simulink model "A3VSM390"  (R2022a)
settings: Solver=ode14x  StartTime=0  StopTime=Sim.tend  FixedStep=0.000125  RelTol=4e-4
values from neighbouring files (symbols this model uses):
  center_line_status = parameterset.center_line_status    [sim3run_390.m]
  ControlSampleTime = 1/8000    (= 0.000125)    [sim3run_390.m]
  k_ring1 = 1    [sim3run_390.m]
  k_ring2 = 1    [sim3run_390.m]
  load_start_factor = 1    [prm3var_390.m]    (also in simu3_826.m = 0.9; simu3_827.m = 0.9)
  lower_line_status = parameterset.lower_line_status    [sim3run_390.m]
  mZC = 3    [sim3run_390.m]
undefined symbols (not defined in the file or in its folder): Event, General, InfBus, Li, parameterset, prm_vsm, pu_vsm, TrG, VSM
libraries: fl_lib x92, nesl_utility x69, ee_lib x36, spsPower3phInstantaneousLib x5, simulink x2, eeTransforms x1
(part 1 of 3)
settings Model: Creator=e2n052  LastModifiedBy=uk062294
settings SolverCC: AlgebraicLoopSolver=TrustRegion
settings DataIOCC: ReturnWorkspaceOutputs=off
settings DebuggingCC: UnconnectedInputMsg=warning  UnconnectedOutputMsg=warning  UnconnectedLineMsg=warning  ArithmeticOperatorsInVariantConditions=warning
settings SFSimCC: SimUseLocalCustomCode=off  CustomCodeUndefinedFunction=UseInterfaceOnly
settings RTWCC: RTWUseLocalCustomCode=off  DLArmComputeVersion=19.05

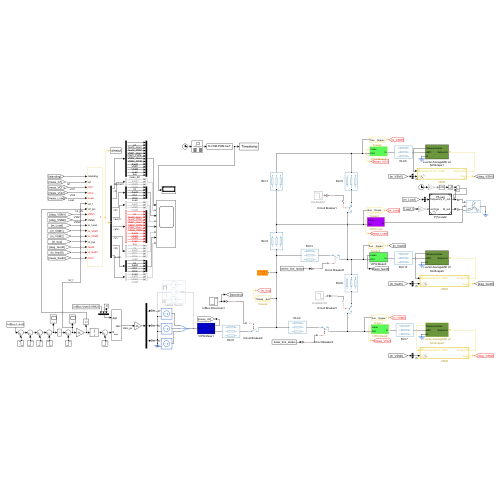
[thumbnail: Simulink's stored preview of the top-level diagram]
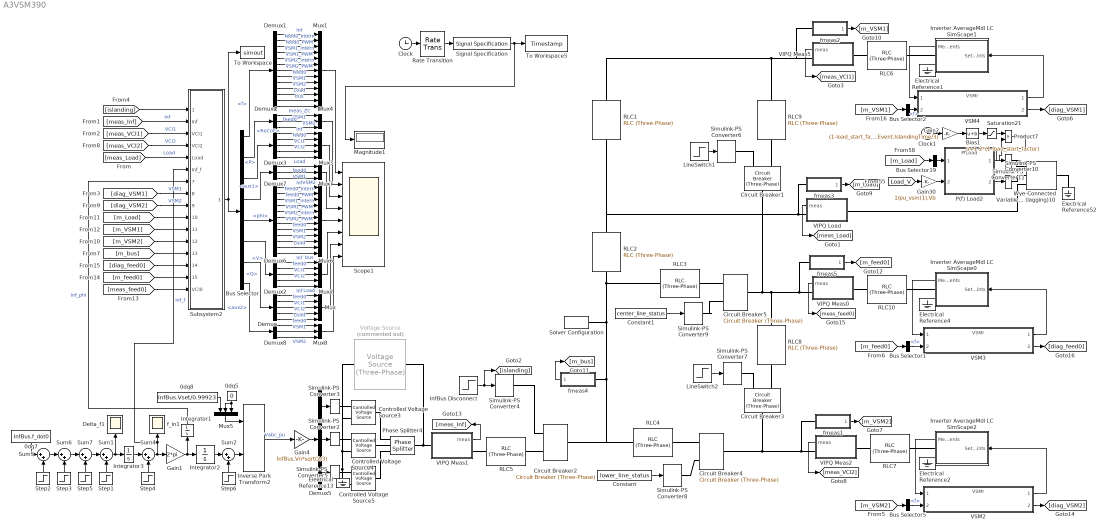
== system A3VSM390 ==
  0dq5 : Constant  Value=0
  0dq7 : Constant  Value=InfBus.f_dot0
  0dq8 : Constant  Value=InfBus.Vset/0.99923
  Bias1 : Bias  Bias=1-2*(1-load_start_factor)  SaturateOnIntegerOverflow=off
  Bus Selector : BusSelector  OutputSignals=f,RoCoF,P,aux1,phi,V,Q,aux2
  Bus Selector1 : BusSelector  OutputSignals=f
  Bus Selector19 : BusSelector  OutputSignals=f  OutputAsBus=on
  Bus Selector2 : BusSelector  OutputSignals=f
  Bus Selector5 : BusSelector  OutputSignals=f
  Circuit Breaker{1,3..5} (4 alike) : ee_lib/Switches & Breakers/Circuit Breaker (Three-Phase)  R_closed=0.0001 Ohm  G_open=1e-6 1/Ohm  threshold=0.5 V  breaker_behavior=ee.enum.switches.breakerBehavior.zeroCrossingEnable
      settings: InternalSimscapePortConfiguration="{\"Bottom\":[],\"Left\":[{\"id\":\"vT\",\"label\":\"vT\",\"type\":\"input\"},{\"id\":\"N1\",\"label\":\"~1\",\"type\":\"foundation.electrical.three_phase\"}],\"Right\":[{\"id\":\"N2\",\"label\":\"~2\",\"type\":\"foundation.electrical.three_phase\"}],\"Top\":[]}"
  Circuit Breaker2 : ee_lib/Switches & Breakers/Circuit Breaker (Three-Phase)  R_closed=0.001 Ohm  G_open=1e-6 1/Ohm  threshold=0.5 V  breaker_behavior=ee.enum.switches.breakerBehavior.zeroCrossingEnable
      settings: InternalSimscapePortConfiguration="{\"Bottom\":[],\"Left\":[{\"id\":\"vT\",\"label\":\"vT\",\"type\":\"input\"},{\"id\":\"N1\",\"label\":\"~1\",\"type\":\"foundation.electrical.three_phase\"}],\"Right\":[{\"id\":\"N2\",\"label\":\"~2\",\"type\":\"foundation.electrical.three_phase\"}],\"Top\":[]}"
  Clock : Clock
  Clock1 : Clock
  Constant : Constant  Value=lower_line_status
  Constant1 : Constant  Value=center_line_status
  Controlled Voltage Source3 : fl_lib/Electrical/Electrical Sources/Controlled Voltage Source
  Controlled Voltage Source4 : fl_lib/Electrical/Electrical Sources/Controlled Voltage Source
  Controlled Voltage Source5 : fl_lib/Electrical/Electrical Sources/Controlled Voltage Source
  Delta_f1 : Scope
  Demux : Demux  Outputs=5
  Demux1 : Demux  Outputs=13
  Demux2 : Demux  Outputs=5
  Demux3 : Demux  Outputs=5
  Demux{4..5,7..8} (4 alike) : Demux  Outputs=3
  Demux6 : Demux  Outputs=12
  Electrical Reference{1..2,4,13,52} (5 alike) : fl_lib/Electrical/Electrical Elements/Electrical Reference
  Gain1 : Gain  Gain=2*pi
  Gain2 : Gain  Gain=(1-load_start_factor)/(parameterset.Event.IslandingTime/3)
  Gain30 : Gain  Gain=1/pu_vsm(1).Vb
  Gain4 : Gain  Gain=InfBus.Vn*sqrt(2/3)
  InfBus Disconnect : Step  Time=Event.IslandingTime  SampleTime=0
  Integrator1 : Integrator  InitialCondition=0+prm_vsm{19,2}  WrappedStateUpperValue=2*pi  WrappedStateLowerValue=0
  Integrator2 : Integrator  InitialCondition=pi/2+prm_vsm{19,2}  WrappedStateUpperValue=2*pi  WrappedStateLowerValue=0
  Integrator3 : Integrator  InitialCondition=InfBus.f_init-InfBus.fn
  Inverse Park Transform2 : eeTransforms/Inverse Park Transform  AxisAlignment=Q-axis  PowerInvariant=off
  Inverter AverageMdl LC SimScape0 : Subsystem  VariantControl=PMXXF33C  mask{L1=prm_vsm{40,3}, R_L1=prm_vsm{43,3}, C1=prm_vsm{42,3}, R_C1=prm_vsm{45,3}}
      mask prompts: L1 "Inductance L1 [H]"; R_L1 "Resistance of L1 [Ohm]"; C1 "Capacitance C1 [F]"; R_C1 "Parallel resistance of C1 [Ohm]"
      mask DialogControl GrpLC Prompt: LC(L)(C)-Filter
  Inverter AverageMdl LC SimScape1 : Subsystem  VariantControl=PMXXF33C  mask{L1=prm_vsm{40,4}, R_L1=prm_vsm{43,4}, C1=prm_vsm{42,4}, R_C1=prm_vsm{45,4}}
      mask prompts: L1 "Inductance L1 [H]"; R_L1 "Resistance of L1 [Ohm]"; C1 "Capacitance C1 [F]"; R_C1 "Parallel resistance of C1 [Ohm]"
      mask DialogControl GrpLC Prompt: LC(L)(C)-Filter
  Inverter AverageMdl LC SimScape2 : Subsystem  VariantControl=PMXXF33C  mask{L1=prm_vsm{40,2}, R_L1=prm_vsm{43,2}, C1=prm_vsm{42,2}, R_C1=prm_vsm{45,2}}
      mask prompts: L1 "Inductance L1 [H]"; R_L1 "Resistance of L1 [Ohm]"; C1 "Capacitance C1 [F]"; R_C1 "Parallel resistance of C1 [Ohm]"
      mask DialogControl GrpLC Prompt: LC(L)(C)-Filter
  "LineSwitch1 " : Step  Time=Event.ring1_switch_time  Before=Event.ring1_switch_direction  After=1-Event.ring1_switch_direction  SampleTime=0
  LineSwitch2 : Step  Time=Event.ring2_switch_time  Before=Event.ring2_switch_direction  After=1-Event.ring2_switch_direction  SampleTime=0
  Magnitude1 : Display
  Mux : Mux  Inputs=5
  Mux1 : Mux  Inputs=13
  Mux2 : Mux  Inputs=5
  Mux3 : Mux  Inputs=5
  Mux{4..5,7..8} (4 alike) : Mux  Inputs=3
  Mux6 : Mux  Inputs=12
  P(f) Load2 : ModelReference  ModelNameDialog=PfLoad.slx  UsingDefaultArgumentValue=0  SimulationMode=Normal  ModelReferenceVersion=11.283
  Phase Splitter4 : ee_lib/Connectors & References/Phase Splitter
  Product7 : Product
  RLC1 : ee_lib/Passive/RLC Assemblies/RLC (Three-Phase)  component_structure=4  R=Li.length*Li.R Ohm  L=Li.length*Li.L H  C=1e-6 F  R_parasitic=1e-6 Ohm  G_parasitic=1e-6 1/Ohm  IL_specify=on  IL_priority=High  IL=[0, 0, 0] A  IL_nominal_specify=off  IL_nominal_unit=A  IL_nominal_value=1  VC_specify=on  VC_priority=High  VC=[0, 0, 0] V  VC_nominal_specify=off  VC_nominal_unit=V  VC_nominal_value=1
      settings: InternalSimscapePortConfiguration="{\"Bottom\":[],\"Left\":[{\"id\":\"N1\",\"label\":\"~1\",\"type\":\"foundation.electrical.three_phase\"}],\"Right\":[{\"id\":\"N2\",\"label\":\"~2\",\"type\":\"foundation.electrical.three_phase\"}],\"Top\":[]}"
  RLC10 : ee_lib/Passive/RLC Assemblies/RLC (Three-Phase)  component_structure=4  R=prm_vsm{44,3} Ohm  L=prm_vsm{41,3} H  C=1e-6 F  R_parasitic=1e-6 Ohm  G_parasitic=1e-6 1/Ohm  IL_specify=on  IL_priority=High  IL=[0, 0, 0] A  IL_nominal_specify=off  IL_nominal_unit=A  IL_nominal_value=1  VC_specify=on  VC_priority=High  VC=[0, 0, 0] V  VC_nominal_specify=off  VC_nominal_unit=V  VC_nominal_value=1
      settings: InternalSimscapePortConfiguration="{\"Bottom\":[],\"Left\":[{\"id\":\"N1\",\"label\":\"~1\",\"type\":\"foundation.electrical.three_phase\"}],\"Right\":[{\"id\":\"N2\",\"label\":\"~2\",\"type\":\"foundation.electrical.three_phase\"}],\"Top\":[]}"
  RLC2 : ee_lib/Passive/RLC Assemblies/RLC (Three-Phase)  component_structure=4  R=Li.length*Li.R Ohm  L=Li.length*Li.L H  C=1e-6 F  R_parasitic=1e-6 Ohm  G_parasitic=1e-6 1/Ohm  IL_specify=on  IL_priority=High  IL=[0, 0, 0] A  IL_nominal_specify=off  IL_nominal_unit=A  IL_nominal_value=1  VC_specify=on  VC_priority=High  VC=[0, 0, 0] V  VC_nominal_specify=off  VC_nominal_unit=V  VC_nominal_value=1
      settings: InternalSimscapePortConfiguration="{\"Bottom\":[],\"Left\":[{\"id\":\"N1\",\"label\":\"~1\",\"type\":\"foundation.electrical.three_phase\"}],\"Right\":[{\"id\":\"N2\",\"label\":\"~2\",\"type\":\"foundation.electrical.three_phase\"}],\"Top\":[]}"
  RLC3 : ee_lib/Passive/RLC Assemblies/RLC (Three-Phase)  component_structure=4  R=2*Li.length*Li.R Ohm  L=2*Li.length*Li.L H  C=1e-6 F  R_parasitic=1e-6 Ohm  G_parasitic=1e-6 1/Ohm  IL_specify=on  IL_priority=High  IL=[0, 0, 0] A  IL_nominal_specify=off  IL_nominal_unit=A  IL_nominal_value=1  VC_specify=on  VC_priority=High  VC=[0, 0, 0] V  VC_nominal_specify=off  VC_nominal_unit=V  VC_nominal_value=1
      settings: InternalSimscapePortConfiguration="{\"Bottom\":[],\"Left\":[{\"id\":\"N1\",\"label\":\"~1\",\"type\":\"foundation.electrical.three_phase\"}],\"Right\":[{\"id\":\"N2\",\"label\":\"~2\",\"type\":\"foundation.electrical.three_phase\"}],\"Top\":[]}"
  RLC4 : ee_lib/Passive/RLC Assemblies/RLC (Three-Phase)  component_structure=4  R=2*Li.length*Li.R Ohm  L=2*Li.length*Li.L H  C=1e-6 F  R_parasitic=1e-6 Ohm  G_parasitic=1e-6 1/Ohm  IL_specify=on  IL_priority=High  IL=[0, 0, 0] A  IL_nominal_specify=off  IL_nominal_unit=A  IL_nominal_value=1  VC_specify=on  VC_priority=High  VC=[0, 0, 0] V  VC_nominal_specify=off  VC_nominal_unit=V  VC_nominal_value=1
      settings: InternalSimscapePortConfiguration="{\"Bottom\":[],\"Left\":[{\"id\":\"N1\",\"label\":\"~1\",\"type\":\"foundation.electrical.three_phase\"}],\"Right\":[{\"id\":\"N2\",\"label\":\"~2\",\"type\":\"foundation.electrical.three_phase\"}],\"Top\":[]}"
  RLC5 : ee_lib/Passive/RLC Assemblies/RLC (Three-Phase)  component_structure=4  R=TrG.R Ohm  L=TrG.L H  C=1e-6 F  R_parasitic=1e-6 Ohm  G_parasitic=1e-6 1/Ohm  IL_specify=on  IL_priority=High  IL=[0, 0, 0] A  IL_nominal_specify=off  IL_nominal_unit=A  IL_nominal_value=1  VC_specify=on  VC_priority=High  VC=[0, 0, 0] V  VC_nominal_specify=off  VC_nominal_unit=V  VC_nominal_value=1
      settings: InternalSimscapePortConfiguration="{\"Bottom\":[],\"Left\":[{\"id\":\"N1\",\"label\":\"~1\",\"type\":\"foundation.electrical.three_phase\"}],\"Right\":[{\"id\":\"N2\",\"label\":\"~2\",\"type\":\"foundation.electrical.three_phase\"}],\"Top\":[]}"
  RLC6 : ee_lib/Passive/RLC Assemblies/RLC (Three-Phase)  component_structure=4  R=prm_vsm{44,4} Ohm  L=prm_vsm{41,4} H  C=1e-6 F  R_parasitic=1e-6 Ohm  G_parasitic=1e-6 1/Ohm  IL_specify=on  IL_priority=High  IL=[0, 0, 0] A  IL_nominal_specify=off  IL_nominal_unit=A  IL_nominal_value=1  VC_specify=on  VC_priority=High  VC=[0, 0, 0] V  VC_nominal_specify=off  VC_nominal_unit=V  VC_nominal_value=1
      settings: InternalSimscapePortConfiguration="{\"Bottom\":[],\"Left\":[{\"id\":\"N1\",\"label\":\"~1\",\"type\":\"foundation.electrical.three_phase\"}],\"Right\":[{\"id\":\"N2\",\"label\":\"~2\",\"type\":\"foundation.electrical.three_phase\"}],\"Top\":[]}"
  RLC7 : ee_lib/Passive/RLC Assemblies/RLC (Three-Phase)  component_structure=4  R=prm_vsm{44,2} Ohm  L=prm_vsm{41,2} H  C=1e-6 F  R_parasitic=1e-6 Ohm  G_parasitic=1e-6 1/Ohm  IL_specify=on  IL_priority=High  IL=[0, 0, 0] A  IL_nominal_specify=off  IL_nominal_unit=A  IL_nominal_value=1  VC_specify=on  VC_priority=High  VC=[0, 0, 0] V  VC_nominal_specify=off  VC_nominal_unit=V  VC_nominal_value=1
      settings: InternalSimscapePortConfiguration="{\"Bottom\":[],\"Left\":[{\"id\":\"N1\",\"label\":\"~1\",\"type\":\"foundation.electrical.three_phase\"}],\"Right\":[{\"id\":\"N2\",\"label\":\"~2\",\"type\":\"foundation.electrical.three_phase\"}],\"Top\":[]}"
  RLC8 : ee_lib/Passive/RLC Assemblies/RLC (Three-Phase)  component_structure=4  R=k_ring2*Li.length*Li.R Ohm  L=k_ring2*Li.length*Li.L H  C=1e-6 F  R_parasitic=1e-6 Ohm  G_parasitic=1e-6 1/Ohm  IL_specify=on  IL_priority=High  IL=[0, 0, 0] A  IL_nominal_specify=off  IL_nominal_unit=A  IL_nominal_value=1  VC_specify=on  VC_priority=High  VC=[0, 0, 0] V  VC_nominal_specify=off  VC_nominal_unit=V  VC_nominal_value=1
      settings: InternalSimscapePortConfiguration="{\"Bottom\":[],\"Left\":[{\"id\":\"N1\",\"label\":\"~1\",\"type\":\"foundation.electrical.three_phase\"}],\"Right\":[{\"id\":\"N2\",\"label\":\"~2\",\"type\":\"foundation.electrical.three_phase\"}],\"Top\":[]}"
  RLC9 : ee_lib/Passive/RLC Assemblies/RLC (Three-Phase)  component_structure=4  R=k_ring1*Li.length*Li.R Ohm  L=k_ring1*Li.length*Li.L H  C=1e-6 F  R_parasitic=1e-6 Ohm  G_parasitic=1e-6 1/Ohm  IL_specify=on  IL_priority=High  IL=[0, 0, 0] A  IL_nominal_specify=off  IL_nominal_unit=A  IL_nominal_value=1  VC_specify=on  VC_priority=High  VC=[0, 0, 0] V  VC_nominal_specify=off  VC_nominal_unit=V  VC_nominal_value=1
      settings: InternalSimscapePortConfiguration="{\"Bottom\":[],\"Left\":[{\"id\":\"N1\",\"label\":\"~1\",\"type\":\"foundation.electrical.three_phase\"}],\"Right\":[{\"id\":\"N2\",\"label\":\"~2\",\"type\":\"foundation.electrical.three_phase\"}],\"Top\":[]}"
  Rate Transition : RateTransition  OutPortSampleTimeOpt=Inherit
  Saturation21 : Saturate  UpperLimit=1  LowerLimit=load_start_factor
  Scope1 : Scope  NumInputPorts=8
  Signal Specification : SignalSpecification  SampleTime=VSM.PWM.tauT
  Simulink-PS Converter{4,6..11} (7 alike) : nesl_utility/Simulink-PS Converter  PhysicalDomain=network_engine_domain  SubClassName=ps_input  LeftPortType=input  RightPortType=output  PseudoPeriodic=off  Frequencies=[]  NoiseDistribution=none  NoiseParameters=[]  Unit=1  AffineConversion=off  FilteringAndDerivatives=zero  SimscapeFilterOrder=1  InputFilterTimeConstant=0.001  UdotUserProvided=1
  Simulink-PS Converter2 : nesl_utility/Simulink-PS Converter  PhysicalDomain=network_engine_domain  SubClassName=ps_input  LeftPortType=input  RightPortType=output  PseudoPeriodic=off  Frequencies=[]  NoiseDistribution=none  NoiseParameters=[]  Unit=V  AffineConversion=off  FilteringAndDerivatives=filter  SimscapeFilterOrder=1  InputFilterTimeConstant=T_PSconv  UdotUserProvided=2
  Simulink-PS Converter3 : nesl_utility/Simulink-PS Converter  PhysicalDomain=network_engine_domain  SubClassName=ps_input  LeftPortType=input  RightPortType=output  PseudoPeriodic=off  Frequencies=[]  NoiseDistribution=none  NoiseParameters=[]  Unit=V  AffineConversion=off  FilteringAndDerivatives=filter  SimscapeFilterOrder=1  InputFilterTimeConstant=T_PSconv  UdotUserProvided=2
  Simulink-PS Converter5 : nesl_utility/Simulink-PS Converter  PhysicalDomain=network_engine_domain  SubClassName=ps_input  LeftPortType=input  RightPortType=output  PseudoPeriodic=off  Frequencies=[]  NoiseDistribution=none  NoiseParameters=[]  Unit=V  AffineConversion=off  FilteringAndDerivatives=filter  SimscapeFilterOrder=1  InputFilterTimeConstant=T_PSconv  UdotUserProvided=2
  Solver Configuration : nesl_utility/Solver Configuration  PhysicalDomain=network_engine_domain  SubClassName=solver  LeftPortType=input  RightPortType=generic  Tones=[]  Harmonics=[]  SimulateNoise=off  Profile=off  UseLocalSampling=off  EnableSwitchedLinearOptims=on  FrequencyDomain=off  UseCCode=off  RelTol=0.001  AbsTol=1e-06  MinStep=1e-09  ToWorkspace=off  RevertToSquareIcSolve=off  NumHomotopyIterations=100  PhasorMode=off  PhasorModeNumHarmonics=1  ConsistencySolver=NEWTON_FTOL  IndexReductionMethod=DerivativeReplacement  DoDC=off  ResidualTolerance=1e-09  ConsistencyTolSource=GLOBAL  ConsistencyAbsTol=0.001  ConsistencyRelTol=0.001  ConsistencyTolFactor=0.001  UseLocalSolver=on  LocalSolverChoice=NE_BACKWARD_EULER_ADVANCER  ResolveIndetEquations=on  FunctionEvalNumThread=1  LocalSolverSampleTime=1/8e3  DoFixedCost=on  MaxNonlinIter=3  MaxModeIter=2  ComputeImpulses=off  ImpulseIterations=2  LinearAlgebra=Sparse  LinearAlgebraNumThread=0  EquationFormulation=NE_TIME_EF  DelaysMemoryBudget=1024  AutomaticFiltering=off  FilteringTimeConstant=0.001  PartitionStorageMethod=AS_NEEDED  PartitionMemoryBudget=1024  PartitionMethod=FAST  MultibodyUseLocalSolver=off  MultibodyLocalSolverChoice=ODE1  MultibodyLocalSolverSampleTime=0.001
  Step1 : Step  Time=InfBus.t_fd4  After=InfBus.f_dot4-InfBus.f_dot3  SampleTime=0
  Step2 : Step  Time=InfBus.t_fd1  After=InfBus.f_dot1-InfBus.f_dot0  SampleTime=0
  Step3 : Step  Time=InfBus.t_fd2  After=InfBus.f_dot2-InfBus.f_dot1  SampleTime=0
  Step4 : Step  Time=InfBus.t_f1  Before=InfBus.fn  After=InfBus.f1  SampleTime=0
  Step5 : Step  Time=InfBus.t_fd3  After=InfBus.f_dot3-InfBus.f_dot2  SampleTime=0
  Step6 : Step  Time=InfBus.t_theta1  After=InfBus.delta_theta1  SampleTime=0
  Subsystem2 : Subsystem
  Sum{1..2,4..7} (6 alike) : Sum  Inputs=|++
  To Workspace : ToWorkspace  VariableName=simout  SampleTime=-1
  To Workspace5 : ToWorkspace  VariableName=Timestamp  SampleTime=-1
  VIPQ Load : Subsystem
  VIPQ Meas0 : Subsystem
  VIPQ Meas1 : Subsystem
  VIPQ Meas2 : Subsystem
  VIPQ Meas5 : Subsystem
  VSM2 : ModelReference  ModelNameDialog=VSMr.slx  UsingDefaultArgumentValue=0  SimulationMode=Normal  ModelReferenceVersion=8.11
  VSM3 : ModelReference  ModelNameDialog=VSMr.slx  UsingDefaultArgumentValue=0  SimulationMode=Normal  ModelReferenceVersion=8.11
  VSM4 : ModelReference  ModelNameDialog=VSMr.slx  UsingDefaultArgumentValue=0  SimulationMode=Normal  ModelReferenceVersion=8.11
  Voltage Source : ee_lib/Sources/Voltage Source (Three-Phase)  Commented=on  vline_rms=InfBus.Vn*InfBus.Vset V  shift=pi/2+VSM.VSM.Phi0-pi/2*0.12 rad  freq=InfBus.fn Hz  impedance_option=0  SShortCircuit=500e6 V*A  XR=10  R=0.01 Ohm  L=3.97e-4 H  harmonic_option=0  harmonic_orders=[5, 7, 11, 13]  harmonic_ratios=[0.1, 0.1, 0.1, 0.1]  G_parasitic=0 1/Ohm  I_specify=off  I_priority=None  I=[ 0 0 0 ] A  I_nominal_specify=off  I_nominal_unit=A  I_nominal_value=1
  Wye-Connected Variable Load (lagging)10 : ee_lib/Passive/RLC Assemblies/Wye-Connected Variable Load (lagging)  VRated=int_sup_vol1 V  FRated=50 Hz  Pmin=10 W  Qmin=10 A*V  G_parasitic=1e-6 1/Ohm  I_specify=off  I_priority=None  I=[0, 0, 0] A  I_nominal_specify=off  I_nominal_unit=A  I_nominal_value=1  Phi_specify=off  Phi_priority=None  Phi=[0, 0, 0] Wb  Phi_nominal_specify=off  Phi_nominal_unit=Wb  Phi_nominal_value=1
      settings: InternalSimscapePortConfiguration="{\"Bottom\":[],\"Left\":[{\"id\":\"P\",\"label\":\"P\",\"type\":\"input\"},{\"id\":\"Q\",\"label\":\"Q\",\"type\":\"input\"},{\"id\":\"N\",\"label\":\"~\",\"type\":\"foundation.electrical.three_phase\"}],\"Right\":[{\"id\":\"n\",\"label\":\"n\",\"type\":\"foundation.electrical.electrical\"}],\"Top\":[]}"
  f_in1 : Scope
  fmeas{1..5} (5 alike) : Subsystem  ReferencedSubsystem=f_meas
  wires:
  InfBus Disconnect/1 -> [islanding], Simulink-PS Converter4/1
  Bus Selector/7 -> Demux/1  "<Q>"
  Bus Selector/3 -> Demux3/1  "<P>"
  Demux3/1 -> Mux3/1  "Inf"
  Demux3/3 -> Mux3/3  "VCI1"
  Demux3/4 -> Mux3/4  "VCI2"
  Bus Selector/6 -> Demux2/1  "<V>"
  Demux2/4 -> Mux2/4  "VCI2"
  Demux2/3 -> Mux2/3  "VCI1"
  Demux2/1 -> Mux2/1  "Inf"
  Bus Selector/1 -> Demux1/1  "<f>"
  Demux1/1 -> Mux1/1  "Inf"
  Demux1/4 -> Mux1/4  "VSM1_intern"
  Demux1/5 -> Mux1/5  "VSM1_PWM"
  Demux/4 -> Mux/4  "VCI2"
  Demux/3 -> Mux/3  "VCI1"
  Demux/1 -> Mux/1  "Inf"
  Inverter AverageMdl LC SimScape1/1(Measurements) -> VSM4/1
  Subsystem2/1(Out5) -> Bus Selector/1, To Workspace/1
  VIPQ Meas5/1(meas) -> [meas_VCI1]
  VIPQ Meas1/1(meas) -> [meas_Inf]
  Clock/1 -> Rate Transition/1
  Sum5/1 -> Sum6/1
  Step2/1 -> Sum5/2
  Step5/1 -> Sum7/2
  Gain4/1 -> Demux5/1
  Demux5/3 -> Simulink-PS Converter5/1
  Demux5/2 -> Simulink-PS Converter2/1
  Mux5/1 -> Inverse Park Transform2/1
  Step3/1 -> Sum6/2
  Inverse Park Transform2/1 -> Gain4/1  "Vabc_pu"
  0dq7/1 -> Sum5/1
  Integrator3/1 -> Sum4/1
  0dq5/1 -> Mux5/2, Mux5/3
  Gain1/1 -> Integrator1/1, Integrator2/1
  Sum6/1 -> Sum7/1
  Step1/1 -> Sum1/2
  Sum7/1 -> Sum1/1
  Sum1/1 -> Integrator3/1, Delta_f1/1
  Demux6/4 -> Mux6/4  "VSM1_intern"
  Demux6/5 -> Mux6/5  "VSM1_PWM"
  Demux6/1 -> Mux6/1  "Inf"
  Bus Selector/5 -> Demux6/1  "<phi>"
  Mux1/1 -> Scope1/1
  Mux6/1 -> Scope1/5
  Mux3/1 -> Scope1/3
  Mux/1 -> Scope1/7
  Mux2/1 -> Scope1/6
  Inverter AverageMdl LC SimScape2/1(Measurements) -> VSM2/1
  VIPQ Meas2/1(meas) -> [meas_VCI2]
  Demux2/5 -> Mux2/5  "Load"
  Demux/5 -> Mux/5  "Load"
  Demux3/5 -> Mux3/5  "Load"
  Demux6/6 -> Mux6/6  "VSM2_intern"
  Demux1/6 -> Mux1/6  "VSM2_intern"
  "LineSwitch1 "/1 -> Simulink-PS Converter6/1
  VSM2/2 -> [diag_VSM2]
  VIPQ Load/1(meas) -> [meas_Load]
  VSM4/2 -> [diag_VSM1]
  Demux1/7 -> Mux1/7  "VSM2_PWM"
  Demux1/9 -> Mux1/9  "VSM1"
  Demux1/10 -> Mux1/10  "VSM2"
  Demux1/11 -> Mux1/11  "Load"
  Demux6/7 -> Mux6/7  "VSM2_PWM"
  Demux6/9 -> Mux6/9  "VSM1"
  Demux6/10 -> Mux6/10  "VSM2"
  [islanding] -> Subsystem2/1(Islanding)
  [meas_Inf] -> Subsystem2/2(Inf)  "Inf"
  [meas_VCI1] -> Subsystem2/3(VCI1)  "VCI1"
  [meas_VCI2] -> Subsystem2/4(VCI2)  "VCI2"
  [meas_Load] -> Subsystem2/5(Load)  "Load"
  Sum4/1 -> Subsystem2/6(Inf_f), f_in1/1, Gain1/1  "Inf_f"
  Integrator1/1 -> Subsystem2/7(Inf_phi)  "Inf_phi"
  [diag_VSM1] -> Subsystem2/8(VSM1)  "VSM1"
  [diag_VSM2] -> Subsystem2/9(VSM2)  "VSM2"
  [m_Load] -> Subsystem2/10(m_Load)
  [m_VSM1] -> Subsystem2/11(m_VSM1)
  Bus Selector/4 -> Demux7/1  "<aux1>"
  Bus Selector/8 -> Demux8/1  "<aux2>"
  0dq8/1 -> Mux5/1
  Demux5/1 -> Simulink-PS Converter3/1
  Integrator2/1 -> Sum2/1
  [m_VSM2] -> Subsystem2/12(m_VSM2)
  Demux1/12 -> Mux1/12  "bus"
  Demux1/13 -> Mux1/13  "meas_ZC"
  Demux6/11 -> Mux6/11  "Load"
  fmeas1/1 -> [m_VSM2]
  fmeas2/1 -> [m_VSM1]
  fmeas4/1 -> [m_bus]
  fmeas3/1 -> [m_Load]
  Demux6/12 -> Mux6/12  "bus"
  [m_bus] -> Subsystem2/13(m_bus)
  Step4/1 -> Sum4/2
  LineSwitch2/1 -> Simulink-PS Converter7/1
  Inverter AverageMdl LC SimScape0/1(Measurements) -> VSM3/1
  VIPQ Meas0/1(meas) -> [meas_feed0]
  fmeas5/1 -> [m_feed0]
  VSM3/2 -> [diag_feed0]
  [m_feed0] -> Subsystem2/15(m_feed0)
  Demux1/8 -> Mux1/8  "feed0"
  Demux1/3 -> Mux1/3  "feed0_PWM"
  Demux1/2 -> Mux1/2  "feed0_intern"
  Demux6/2 -> Mux6/2  "feed0_intern"
  Demux6/3 -> Mux6/3  "feed0_PWM"
  Demux6/8 -> Mux6/8  "feed0"
  Demux3/2 -> Mux3/2  "feed0"
  Demux/2 -> Mux/2  "feed0"
  Demux2/2 -> Mux2/2  "feed0"
  [diag_feed0] -> Subsystem2/14(feed0)
  [meas_feed0] -> Subsystem2/16(VCI0)
  Demux7/1 -> Mux7/1  "feed0"
  Demux7/2 -> Mux7/2  "VSM1"
  Demux7/3 -> Mux7/3  "VSM2"
  Mux7/1 -> Scope1/4
  Demux8/1 -> Mux8/1  "feed0"
  Demux8/3 -> Mux8/3  "VSM2"
  Demux8/2 -> Mux8/2  "VSM1"
  Mux8/1 -> Scope1/8
  Rate Transition/1 -> Signal Specification/1
  Signal Specification/1 -> Magnitude1/1, To Workspace5/1
  Constant/1 -> Simulink-PS Converter8/1
  Constant1/1 -> Simulink-PS Converter9/1
  Gain30/1 -> P(f) Load2/2
  Product7/1 -> Simulink-PS Converter11/1
  Bus Selector19/1 -> P(f) Load2/1
  P(f) Load2/2 -> Simulink-PS Converter10/1
  [m_Load] -> Bus Selector19/1
  [m_VSM2] -> Bus Selector5/1
  Bus Selector5/1 -> VSM2/2  "<f>"
  [m_feed0] -> Bus Selector1/1
  Bus Selector1/1 -> VSM3/2  "<f>"
  Bus Selector2/1 -> VSM4/2  "<f>"
  [m_VSM1] -> Bus Selector2/1
  VSM2/1 -> Inverter AverageMdl LC SimScape2/1(Setpoints)
  VSM3/1 -> Inverter AverageMdl LC SimScape0/1(Setpoints)
  VSM4/1 -> Inverter AverageMdl LC SimScape1/1(Setpoints)
  [Load_V] -> Gain30/1
  Clock1/1 -> Gain2/1
  P(f) Load2/1 -> Product7/2
  Saturation21/1 -> Product7/1
  Step6/1 -> Sum2/2
  Sum2/1 -> Inverse Park Transform2/2
  Mux4/1 -> Scope1/2
  Demux4/2 -> Mux4/2  "VSM1"
  Demux4/1 -> Mux4/1  "feed0"
  Bus Selector/2 -> Demux4/1  "<RoCoF>"
  Demux4/3 -> Mux4/3  "VSM2"
  Bias1/1 -> Saturation21/1
  Gain2/1 -> Bias1/1
  connections:
  Circuit Breaker2/LConn1 -- Simulink-PS Converter4/RConn1
  RLC5/LConn1 -- VIPQ Meas1/RConn1
  Inverter AverageMdl LC SimScape1/RConn2 -- Electrical Reference1/LConn1
  Simulink-PS Converter3/RConn1 -- Controlled Voltage Source3/RConn1
  Phase Splitter4/RConn2 -- Controlled Voltage Source4/LConn1
  Simulink-PS Converter5/RConn1 -- Controlled Voltage Source5/RConn1
  Phase Splitter4/RConn1 -- Controlled Voltage Source3/LConn1
  Phase Splitter4/RConn3 -- Controlled Voltage Source5/LConn1
  VIPQ Meas2/LConn1 -- RLC7/LConn1
  fmeas4/LConn1 -- RLC4/RConn1 -- Circuit Breaker2/RConn1 -- Solver Configuration/RConn1 -- RLC3/RConn1 -- RLC2/RConn1
  Circuit Breaker1/LConn1 -- Simulink-PS Converter6/RConn1
  Circuit Breaker2/LConn2 -- RLC5/RConn1
  RLC6/RConn1 -- Inverter AverageMdl LC SimScape1/RConn1
  Simulink-PS Converter2/RConn1 -- Controlled Voltage Source4/RConn1
  Electrical Reference13/LConn1 -- Controlled Voltage Source5/RConn2 -- Voltage Source/LConn1 -- Controlled Voltage Source3/RConn2 -- Controlled Voltage Source4/RConn2
  Inverter AverageMdl LC SimScape2/RConn2 -- Electrical Reference2/LConn1
  VIPQ Meas5/LConn1 -- RLC6/LConn1
  RLC7/RConn1 -- Inverter AverageMdl LC SimScape2/RConn1
  RLC2/LConn1 -- RLC1/RConn1 -- fmeas3/LConn1 -- VIPQ Load/RConn1
  VIPQ Meas0/RConn1 -- RLC8/LConn1 -- Circuit Breaker1/RConn1 -- Circuit Breaker5/RConn1 -- fmeas5/LConn1
  VIPQ Meas1/LConn1 -- Voltage Source/RConn1 -- Phase Splitter4/LConn1
  VIPQ Meas5/RConn1 -- fmeas2/LConn1 -- RLC9/LConn1 -- RLC1/LConn1
  Circuit Breaker3/LConn1 -- Simulink-PS Converter7/RConn1
  Circuit Breaker4/RConn1 -- Circuit Breaker3/RConn1 -- fmeas1/LConn1 -- VIPQ Meas2/RConn1
  RLC10/RConn1 -- Inverter AverageMdl LC SimScape0/RConn1
  VIPQ Meas0/LConn1 -- RLC10/LConn1
  Inverter AverageMdl LC SimScape0/RConn2 -- Electrical Reference4/LConn1
  RLC4/LConn1 -- Circuit Breaker4/LConn2
  Simulink-PS Converter8/RConn1 -- Circuit Breaker4/LConn1
  RLC3/LConn1 -- Circuit Breaker5/LConn2
  Simulink-PS Converter9/RConn1 -- Circuit Breaker5/LConn1
  RLC8/RConn1 -- Circuit Breaker3/LConn2
  RLC9/RConn1 -- Circuit Breaker1/LConn2
  VIPQ Load/LConn1 -- Wye-Connected Variable Load (lagging)10/LConn3
  Wye-Connected Variable Load (lagging)10/RConn1 -- Electrical Reference52/LConn1
  Wye-Connected Variable Load (lagging)10/LConn2 -- Simulink-PS Converter10/RConn1
  Simulink-PS Converter11/RConn1 -- Wye-Connected Variable Load (lagging)10/LConn1

== system A3VSM390/Inverter AverageMdl LC SimScape0 ==
  Setpoints : Inport
  Bus Creator : BusCreator  Inputs=1
  Bus Selector : BusSelector  OutputSignals=Inv1
  Modul F30 fixed DC voltage Average SimScape : Subsystem  mask{L1=L1, R_L1=R_L1, C1=C1, R_C1=R_C1}
      mask prompts: L1 "Inductance L1 [H]"; R_L1 "Resistance of L1 [Ohm]"; C1 "Capacitance C1 [F]"; R_C1 "Parallel resistance of C1 [Ohm]"
      mask DialogControl GrpLoad Prompt: Triphase
      mask DialogControl LC Prompt: LC(L)(C)
      mask DialogControl GrpLC Prompt: LC(L)(C)-Filter
  ABC : PMIOPort  Side=Right
  N : PMIOPort  Port=2  Side=Right
  Measurements : Outport  VectorParamsAs1DForOutWhenUnconnected=off
  wires:
  Modul F30 fixed DC voltage Average SimScape/1(meas) -> Bus Creator/1  "Inv1"
  Bus Creator/1 -> Measurements/1
  Bus Selector/1 -> Modul F30 fixed DC voltage Average SimScape/1(ctrl)  "<Inv1>"
  Setpoints/1 -> Bus Selector/1
  connections:
  N/RConn1 -- Modul F30 fixed DC voltage Average SimScape/LConn1
  ABC/RConn1 -- Modul F30 fixed DC voltage Average SimScape/RConn1

== system A3VSM390/Inverter AverageMdl LC SimScape1 ==
  Setpoints : Inport
  Bus Creator : BusCreator  Inputs=1
  Bus Selector : BusSelector  OutputSignals=Inv1
  Modul F30 fixed DC voltage Average SimScape : Subsystem  mask{L1=L1, R_L1=R_L1, C1=C1, R_C1=R_C1}
      mask prompts: L1 "Inductance L1 [H]"; R_L1 "Resistance of L1 [Ohm]"; C1 "Capacitance C1 [F]"; R_C1 "Parallel resistance of C1 [Ohm]"
      mask DialogControl GrpLoad Prompt: Triphase
      mask DialogControl LC Prompt: LC(L)(C)
      mask DialogControl GrpLC Prompt: LC(L)(C)-Filter
  ABC : PMIOPort  Side=Right
  N : PMIOPort  Port=2  Side=Right
  Measurements : Outport  VectorParamsAs1DForOutWhenUnconnected=off
  wires:
  Modul F30 fixed DC voltage Average SimScape/1(meas) -> Bus Creator/1  "Inv1"
  Bus Creator/1 -> Measurements/1
  Bus Selector/1 -> Modul F30 fixed DC voltage Average SimScape/1(ctrl)  "<Inv1>"
  Setpoints/1 -> Bus Selector/1
  connections:
  N/RConn1 -- Modul F30 fixed DC voltage Average SimScape/LConn1
  ABC/RConn1 -- Modul F30 fixed DC voltage Average SimScape/RConn1

== system A3VSM390/Inverter AverageMdl LC SimScape2 ==
  Setpoints : Inport
  Bus Creator : BusCreator  Inputs=1
  Bus Selector : BusSelector  OutputSignals=Inv1
  Modul F30 fixed DC voltage Average SimScape : Subsystem  mask{L1=L1, R_L1=R_L1, C1=C1, R_C1=R_C1}
      mask prompts: L1 "Inductance L1 [H]"; R_L1 "Resistance of L1 [Ohm]"; C1 "Capacitance C1 [F]"; R_C1 "Parallel resistance of C1 [Ohm]"
      mask DialogControl GrpLoad Prompt: Triphase
      mask DialogControl LC Prompt: LC(L)(C)
      mask DialogControl GrpLC Prompt: LC(L)(C)-Filter
  ABC : PMIOPort  Side=Right
  N : PMIOPort  Port=2  Side=Right
  Measurements : Outport  VectorParamsAs1DForOutWhenUnconnected=off
  wires:
  Modul F30 fixed DC voltage Average SimScape/1(meas) -> Bus Creator/1  "Inv1"
  Bus Creator/1 -> Measurements/1
  Bus Selector/1 -> Modul F30 fixed DC voltage Average SimScape/1(ctrl)  "<Inv1>"
  Setpoints/1 -> Bus Selector/1
  connections:
  N/RConn1 -- Modul F30 fixed DC voltage Average SimScape/LConn1
  ABC/RConn1 -- Modul F30 fixed DC voltage Average SimScape/RConn1

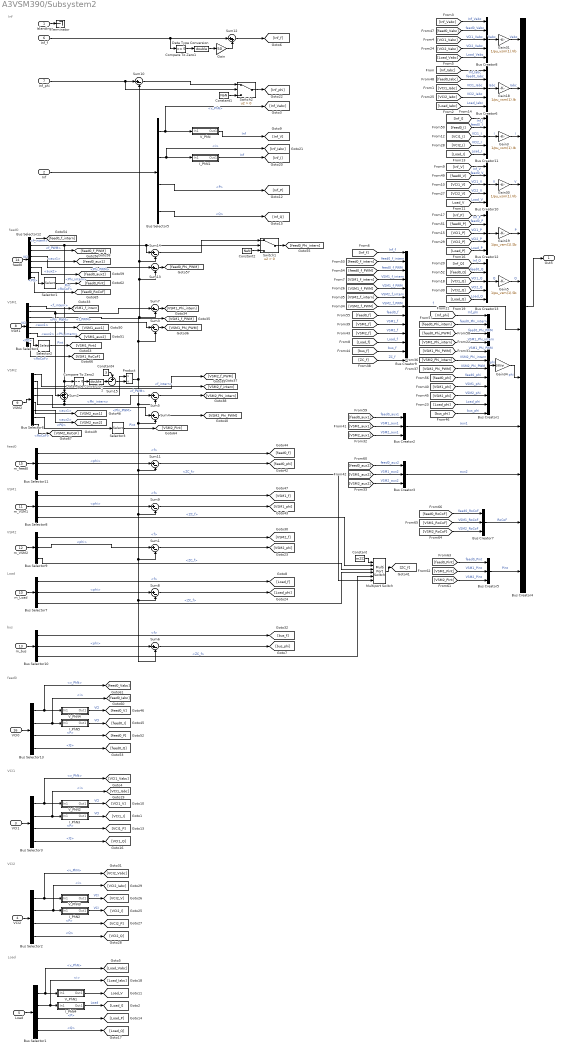
== system A3VSM390/Subsystem2 ==
  note: Load
  note: Inf
  note: VSM1
  note: Load
  note: VSM2
  note: VCI1
  note: VCI2
  note: VSM1
  note: VSM2
  note: bus
  note: feed0
  note: feed0
  note: feed0
  Islanding : Inport
  Inf : Inport  Port=2
  VCI1 : Inport  Port=3
  VCI2 : Inport  Port=4
  Load : Inport  Port=5
  Inf_f : Inport  Port=6
  Inf_phi : Inport  Port=7
  VSM1 : Inport  Port=8
  VSM2 : Inport  Port=9
  m_Load : Inport  Port=10
  m_VSM1 : Inport  Port=11
  m_VSM2 : Inport  Port=12
  m_bus : Inport  Port=13
  feed0 : Inport  Port=14
  m_feed0 : Inport  Port=15
  VCI0 : Inport  Port=16
  Bus Creator1 : BusCreator  Inputs=12
  Bus Creator{6,8,10..13} (6 alike) : BusCreator  Inputs=5
  Bus Creator{2..3,5,7} (4 alike) : BusCreator  Inputs=3
  Bus Creator4 : BusCreator  Inputs=12
  Bus Creator9 : BusCreator  Inputs=13
  Bus Selector{1..3,5,13} (5 alike) : BusSelector  OutputSignals=v_PhN,i,P,Q
  Bus Selector{7..11} (5 alike) : BusSelector  OutputSignals=f,phi,ZC_f
  Bus Selector12 : BusSelector  OutputSignals=Inv1.ctrlDiag.f_intern,Inv1.ctrlDiag.Phi_intern,Inv1.ctrlDiag.f_PWM,Inv1.ctrlDiag.Phi_PWM,Inv1.ctrlDiag.aux1,Inv1.ctrlDiag.aux2,Inv1.measDiag.PQ,Inv1.ctrlDiag.RoCoF
  Bus Selector4 : BusSelector  OutputSignals=Inv1.ctrlDiag.f_intern,Inv1.ctrlDiag.Phi_intern,Inv1.ctrlDiag.f_PWM,Inv1.ctrlDiag.Phi_PWM,Inv1.ctrlDiag.aux1,Inv1.ctrlDiag.aux2,Inv1.measDiag.PQ,Inv1.ctrlDiag.RoCoF
  Bus Selector6 : BusSelector  OutputSignals=Inv1.ctrlDiag.f_intern,Inv1.ctrlDiag.Phi_intern,Inv1.ctrlDiag.f_PWM,Inv1.ctrlDiag.Phi_PWM,Inv1.ctrlDiag.aux1,Inv1.ctrlDiag.aux2,Inv1.measDiag.PQ,Inv1.ctrlDiag.RoCoF
  Compare To Zero1 : simulink/Logic and Bit Operations/Compare To Zero  relop===  OutDataTypeStr=boolean
  Compare To Zero2 : simulink/Logic and Bit Operations/Compare To Zero  relop===  OutDataTypeStr=boolean
  Constant : Constant  Value=mZC
  Constant1 : Constant  Value=NaN
  Constant2 : Constant  Value=NaN
  Constant4 : Constant  Value=3
  Data Type Conversion : DataTypeConversion  OutDataTypeStr=double  SaturateOnIntegerOverflow=off  RndMeth=Floor
  Data Type Conversion1 : DataTypeConversion  OutDataTypeStr=double  SaturateOnIntegerOverflow=off  RndMeth=Floor
  Gain : Gain  Gain=50
  Gain18 : Gain  Gain=1/pu_vsm(1).Ib
  Gain19 : Gain  Gain=1/pu_vsm(1).Sb
  Gain3 : Gain  Gain=1/pu_vsm(1).Ib
  Gain30 : Gain  Gain=1/pu_vsm(1).Vb
  Gain31 : Gain  Gain=1/pu_vsm(1).Vb
  Gain34 : Gain  Gain=180/pi
  Gain5 : Gain  Gain=1/pu_vsm(1).Sb
  I_PhN1 : Subsystem
  I_PhN2 : Subsystem
  I_PhN3 : Subsystem
  I_PhN4 : Subsystem
  I_PhN5 : Subsystem
  Multiport Switch : MultiPortSwitch  Inputs=5  SaturateOnIntegerOverflow=off  InputSameDT=off
  Product : Product  Inputs=*/
  Selector1 : Selector  InputPortWidth=2  IndexOptions=Index vector (dialog)  Indices=1  OutputSizes=1
  Selector2 : Selector  InputPortWidth=2  IndexOptions=Index vector (dialog)  Indices=1  OutputSizes=1
  Selector3 : Selector  InputPortWidth=2  IndexOptions=Index vector (dialog)  Indices=1  OutputSizes=1
  Sum{1,3..11,13..14} (12 alike) : Sum  Inputs=|+-
  Sum12 : Sum  Inputs=|++
  Sum15 : Sum  Inputs=+-|
  Sum2 : Sum  Inputs=+++
  Switch1 : Switch  Criteria=u2 > Threshold  SaturateOnIntegerOverflow=off  InputSameDT=off
  Switch2 : Switch  Criteria=u2 > Threshold  SaturateOnIntegerOverflow=off  InputSameDT=off
  Terminator : Terminator
  V_PhN : Subsystem
  V_PhN1 : Subsystem
  V_PhN2 : Subsystem
  V_PhN3 : Subsystem
  V_PhN4 : Subsystem
  Out5 : Outport  VectorParamsAs1DForOutWhenUnconnected=off
  tag scope: Load_V=global
  wires:
  Bus Creator4/1 -> Out5/1
  Inf/1 -> Bus Selector5/1
  Gain19/1 -> Bus Creator4/5  "P"
  Gain5/1 -> Bus Creator4/6  "Q"
  Bus Selector5/1 -> [Inf_Vabc], V_PhN/1(In1)  "<v_PhN>"
  Bus Selector5/4 -> [Inf_Q]  "<Q>"
  Gain30/1 -> Bus Creator4/4  "V"
  Bus Selector5/3 -> [Inf_P]  "<P>"
  V_PhN/1(Out1) -> [Inf_V]  "Inf"
  Gain31/1 -> Bus Creator4/1  "Vabc"
  Bus Creator11/1 -> Gain3/1  "I"
  [Inf_Iabc] -> Bus Creator6/1  "Inf_Iabc"
  [VCI1_Iabc] -> Bus Creator6/3  "VCI1_Iabc"
  [Load_Iabc] -> Bus Creator6/5  "Load_Iabc"
  [Load_Vabc] -> Bus Creator8/5  "Load_Vabc"
  [VCI1_Vabc] -> Bus Creator8/3  "VCI1_Vabc"
  [Inf_Vabc] -> Bus Creator8/1  "Inf_Vabc"
  [VCI1_V] -> Bus Creator10/3  "VCI1_V"
  [Inf_V] -> Bus Creator10/1  "Inf_V"
  [Inf_I] -> Bus Creator11/1  "Inf_I"
  [VCI1_I] -> Bus Creator11/3  "VCI1_I"
  [VCI1_P] -> Bus Creator12/3  "VCI1_P"
  [Inf_P] -> Bus Creator12/1  "Inf_P"
  [Inf_Q] -> Bus Creator13/1  "Inf_Q"
  [VCI1_Q] -> Bus Creator13/3  "VCI1_Q"
  Gain18/1 -> Bus Creator4/2  "Iabc"
  VSM1/1 -> Bus Selector4/1  "VCI"
  I_PhN1/1(Out1) -> [Inf_I]  "Inf"
  Bus Selector5/2 -> [Inf_Iabc], I_PhN1/1(In1)  "<i>"
  [VSM1_Phi_intern] -> Bus Creator1/4  "VSM1_Phi_intern"
  [VCI2_Vabc] -> Bus Creator8/4  "VCI2_Vabc"
  [VCI2_Iabc] -> Bus Creator6/4  "VCI2_Iabc"
  [Load_V] -> Bus Creator10/5  "Load_V"
  [VCI2_V] -> Bus Creator10/4  "VCI2_V"
  [Load_I] -> Bus Creator11/5  "Load_I"
  [VCI2_I] -> Bus Creator11/4  "VCI2_I"
  [Load_P] -> Bus Creator12/5  "Load_P"
  [VCI2_P] -> Bus Creator12/4  "VCI2_P"
  [Load_Q] -> Bus Creator13/5  "Load_Q"
  [VCI2_Q] -> Bus Creator13/4  "VCI2_Q"
  [VSM1_Phi_PWM] -> Bus Creator1/5  "VSM1_Phi_PWM"
  Bus Creator10/1 -> Gain30/1  "V"
  Bus Creator8/1 -> Gain31/1  "Vabc"
  Bus Creator12/1 -> Gain19/1
  Bus Creator13/1 -> Gain5/1  "Q"
  Bus Creator6/1 -> Gain18/1  "Iabc"
  Gain3/1 -> Bus Creator4/3  "I"
  Bus Selector3/2 -> I_PhN3/1(In1), [VCI1_Iabc]  "<i>"
  Bus Selector3/3 -> [VCI1_P]  "<P>"
  VCI1/1 -> Bus Selector3/1
  Bus Selector3/1 -> [VCI1_Vabc], V_PhN2/1(In1)  "<v_PhN>"
  V_PhN2/1(Out1) -> [VCI1_V]  "VCI"
  Bus Selector3/4 -> [VCI1_Q]  "<Q>"
  I_PhN3/1(Out1) -> [VCI1_I]  "VCI"
  VCI2/1 -> Bus Selector2/1
  Bus Selector2/2 -> [VCI2_Iabc], I_PhN2/1(In1)  "<i>"
  V_PhN3/1(Out1) -> [VCI2_V]  "VCI"
  Bus Selector2/1 -> V_PhN3/1(In1), [VCI2_Vabc]  "<v_PhN>"
  I_PhN2/1(Out1) -> [VCI2_I]  "VCI"
  Bus Selector2/4 -> [VCI2_Q]  "<Q>"
  Bus Selector2/3 -> [VCI2_P]  "<P>"
  Bus Selector1/4 -> [Load_Q]  "<Q>"
  I_PhN4/1(Out1) -> [Load_I]  "Load"
  Bus Selector1/1 -> V_PhN1/1(In1), [Load_Vabc]  "<v_PhN>"
  Load/1 -> Bus Selector1/1
  Bus Selector1/2 -> [Load_Iabc], I_PhN4/1(In1)  "<i>"
  Bus Selector1/3 -> [Load_P]  "<P>"
  Bus Selector4/1 -> [VSM1_f_intern]  "<f_intern>"
  Bus Selector4/3 -> [VSM1_f_PWM]  "<f_PWM>"
  Bus Creator2/1 -> Bus Creator4/9  "aux1"
  Bus Selector6/1 -> [VSM2_f_intern]  "<f_intern>"
  VSM2/1 -> Bus Selector6/1
  Bus Selector6/2 -> Sum5/1, Sum2/3  "<Phi_intern>"
  Bus Selector6/3 -> [VSM2_f_PWM]  "<f_PWM>"
  [VSM2_Phi_PWM] -> Bus Creator1/7  "VSM2_Phi_PWM"
  [VSM2_Phi_intern] -> Bus Creator1/6  "VSM2_Phi_intern"
  Sum3/1 -> [VSM1_Phi_PWM]
  Bus Selector4/4 -> Sum3/1  "<Phi_PWM>"
  Bus Selector6/4 -> Sum4/1  "<Phi_PWM>"
  Sum4/1 -> [VSM2_Phi_PWM]
  Sum5/1 -> [VSM2_Phi_intern]
  Sum7/1 -> [VSM1_Phi_intern]
  Bus Selector4/2 -> Sum2/2, Sum7/1  "<Phi_intern>"
  Gain34/1 -> Bus Creator4/8  "phi"
  Bus Creator1/1 -> Gain34/1  "phi"
  Sum8/1 -> [Load_phi]
  Bus Selector7/1 -> [Load_f]  "<f>"
  Bus Selector7/2 -> Sum8/1  "<phi>"
  m_Load/1 -> Bus Selector7/1
  Bus Selector8/1 -> [VSM1_f]  "<f>"
  Sum9/1 -> [VSM1_phi]
  m_VSM1/1 -> Bus Selector8/1
  Bus Selector6/5 -> [VSM2_aux1]  "<aux1>"
  Bus Selector6/6 -> [VSM2_aux2]  "<aux2>"
  Bus Selector4/5 -> [VSM1_aux1]  "<aux1>"
  Bus Selector4/6 -> [VSM1_aux2]  "<aux2>"
  Bus Creator3/1 -> Bus Creator4/10  "aux2"
  Bus Selector9/1 -> [VSM2_f]  "<f>"
  Sum1/1 -> [VSM2_phi]
  m_VSM2/1 -> Bus Selector9/1
  Bus Selector9/2 -> Sum1/1  "<phi>"
  Bus Selector9/3 -> Multiport Switch/3  "<ZC_f>"
  Bus Selector8/2 -> Sum9/1  "<phi>"
  Bus Selector10/1 -> [bus_f]  "<f>"
  Sum6/1 -> [bus_phi]
  m_bus/1 -> Bus Selector10/1
  Bus Selector10/2 -> Sum6/1  "<phi>"
  [ZC_f] -> Bus Creator9/13  "ZC_f"
  [Load_f] -> Bus Creator9/11  "Load_f"
  [VSM1_f] -> Bus Creator9/9  "VSM1_f"
  [VSM2_f] -> Bus Creator9/10  "VSM2_f"
  [bus_f] -> Bus Creator9/12  "bus_f"
  Constant/1 -> Multiport Switch/1
  Multiport Switch/1 -> [ZC_f]
  Bus Selector8/3 -> Multiport Switch/2  "<ZC_f>"
  Bus Selector7/3 -> Multiport Switch/4  "<ZC_f>"
  Bus Selector10/3 -> Multiport Switch/5  "<ZC_f>"
  Bus Selector12/2 -> Compare To Zero2/1, Sum2/1, Sum14/1, Switch1/2  "<Phi_intern>"
  Sum14/1 -> Switch1/1
  Bus Selector12/1 -> [feed0_f_intern]  "<f_intern>"
  Sum13/1 -> [feed0_Phi_PWM]
  Bus Selector12/6 -> [feed0_aux2]  "<aux2>"
  feed0/1 -> Bus Selector12/1  "VCI"
  Product/1 -> Sum10/2, Sum14/2, Sum13/2, Sum7/2, Sum3/2, Sum6/2, Sum8/2, Sum1/2, Sum9/2, Sum11/2, Sum4/2, Sum5/2
  Bus Selector12/4 -> Sum13/1  "<Phi_PWM>"
  Bus Selector12/5 -> [feed0_aux1]  "<aux1>"
  Bus Selector12/3 -> [feed0_f_PWM]  "<f_PWM>"
  m_feed0/1 -> Bus Selector11/1
  Sum11/1 -> [feed0_phi]
  Bus Selector11/2 -> Sum11/1  "<phi>"
  Bus Selector11/1 -> [feed0_f]  "<f>"
  Bus Selector13/3 -> [feed0_P]  "<P>"
  VCI0/1 -> Bus Selector13/1
  Bus Selector13/4 -> [feed0_Q]  "<Q>"
  I_PhN5/1(Out1) -> [feed0_I]  "VCI"
  Bus Selector13/1 -> [feed0_Vabc], V_PhN4/1(In1)  "<v_PhN>"
  V_PhN4/1(Out1) -> [feed0_V]  "VCI"
  Bus Selector13/2 -> I_PhN5/1(In1), [feed0_Iabc]  "<i>"
  [feed0_Vabc] -> Bus Creator8/2  "feed0_Vabc"
  [feed0_Iabc] -> Bus Creator6/2  "feed0_Iabc"
  [feed0_V] -> Bus Creator10/2  "feed0_V"
  [feed0_I] -> Bus Creator11/2  "feed0_I"
  [feed0_P] -> Bus Creator12/2  "feed0_P"
  [feed0_Q] -> Bus Creator13/2  "feed0_Q"
  Bus Creator9/1 -> Bus Creator4/7  "f"
  [Inf_f] -> Bus Creator9/1  "Inf_f"
  [feed0_f_intern] -> Bus Creator9/2  "feed0_f_intern"
  [feed0_f_PWM] -> Bus Creator9/3  "feed0_f_PWM"
  [VSM2_f_PWM] -> Bus Creator9/7  "VSM2_f_PWM"
  [VSM2_f_intern] -> Bus Creator9/6  "VSM2_f_intern"
  [VSM1_f_intern] -> Bus Creator9/4  "VSM1_f_intern"
  [VSM1_f_PWM] -> Bus Creator9/5  "VSM1_f_PWM"
  [feed0_f] -> Bus Creator9/8  "feed0_f"
  [bus_phi] -> Bus Creator1/12  "bus_phi"
  [VSM2_phi] -> Bus Creator1/10  "VSM2_phi"
  [Load_phi] -> Bus Creator1/11  "Load_phi"
  [VSM1_phi] -> Bus Creator1/9  "VSM1_phi"
  [feed0_phi] -> Bus Creator1/8  "feed0_phi"
  [Inf_phi] -> Bus Creator1/1  "Inf_phi"
  [feed0_Phi_PWM] -> Bus Creator1/3  "feed0_Phi_PWM"
  [feed0_Phi_intern] -> Bus Creator1/2  "feed0_Phi_intern"
  [VSM1_aux1] -> Bus Creator2/2  "VSM1_aux1"
  [VSM2_aux1] -> Bus Creator2/3  "VSM2_aux1"
  [feed0_aux1] -> Bus Creator2/1  "feed0_aux1"
  [VSM1_aux2] -> Bus Creator3/2  "VSM1_aux2"
  [VSM2_aux2] -> Bus Creator3/3  "VSM2_aux2"
  [feed0_aux2] -> Bus Creator3/1  "feed0_aux2"
  Bus Selector11/3 -> Multiport Switch/6  "<ZC_f>"
  Sum12/1 -> [Inf_f]
  Sum2/1 -> Product/1
  Sum15/1 -> Product/2
  Constant2/1 -> Switch1/3
  Switch1/1 -> [feed0_Phi_intern]
  Compare To Zero1/1 -> Data Type Conversion/1
  Data Type Conversion/1 -> Gain/1
  Inf_f/1 -> Compare To Zero1/1, Sum12/1
  Gain/1 -> Sum12/2
  Compare To Zero2/1 -> Data Type Conversion1/1
  Data Type Conversion1/1 -> Sum15/2
  Constant4/1 -> Sum15/1
  Switch2/1 -> [Inf_phi]
  Inf_phi/1 -> Switch2/2, Sum10/1
  Sum10/1 -> Switch2/1
  Islanding/1 -> Terminator/1
  Constant1/1 -> Switch2/3
  V_PhN1/1(Out1) -> [Load_V]
  Bus Selector12/7 -> Selector1/1  "<PQ>"
  Selector1/1 -> [feed0_Pint]  "Pint"
  Bus Creator5/1 -> Bus Creator4/12  "Pint"
  [feed0_Pint] -> Bus Creator5/1  "feed0_Pint"
  [VSM1_Pint] -> Bus Creator5/2  "VSM1_Pint"
  [VSM2_Pint] -> Bus Creator5/3  "VSM2_Pint"
  Bus Selector4/7 -> Selector2/1  "<PQ>"
  Selector2/1 -> [VSM1_Pint]  "Pint"
  Selector3/1 -> [VSM2_Pint]  "Pint"
  Bus Selector6/7 -> Selector3/1  "<PQ>"
  Bus Selector12/8 -> [feed0_RoCoF]  "<RoCoF>"
  [VSM2_RoCoF] -> Bus Creator7/3  "VSM2_RoCoF"
  [VSM1_RoCoF] -> Bus Creator7/2  "VSM1_RoCoF"
  Bus Creator7/1 -> Bus Creator4/11  "RoCoF"
  [feed0_RoCoF] -> Bus Creator7/1  "feed0_RoCoF"
  Bus Selector4/8 -> [VSM1_RoCoF]  "<RoCoF>"
  Bus Selector6/8 -> [VSM2_RoCoF]  "<RoCoF>"

== system A3VSM390/VIPQ Load ==
  note: 2
  Bus Creator : BusCreator  Inputs=4
  Current Sensor : ee_lib/Sensors & Transducers/Current Sensor (Three-Phase)
  Grounded Neutral : ee_lib/Connectors & References/Grounded Neutral (Three-Phase)
  PS-Simulink Converter : nesl_utility/PS-Simulink Converter  PhysicalDomain=network_engine_domain  SubClassName=ps_output  LeftPortType=input  RightPortType=output  PseudoPeriodic=off  Frequencies=[]  VectorFormat=1-D array  Unit=1  AffineConversion=off
  PS-Simulink Converter1 : nesl_utility/PS-Simulink Converter  PhysicalDomain=network_engine_domain  SubClassName=ps_output  LeftPortType=input  RightPortType=output  PseudoPeriodic=off  Frequencies=[]  VectorFormat=1-D array  Unit=1  AffineConversion=off
  Phase Voltage Sensor : ee_lib/Sensors & Transducers/Phase Voltage Sensor (Three-Phase)
  "Power (3ph, Instantaneous)" : spsPower3phInstantaneousLib/Power (3ph, Instantaneous)
  In : PMIOPort  Side=Left
  Out : PMIOPort  Port=2  Side=Right
  meas : Outport  VectorParamsAs1DForOutWhenUnconnected=off
  wires:
  Bus Creator/1 -> meas/1
  "Power (3ph, Instantaneous)"/2 -> Bus Creator/4  "Q"
  "Power (3ph, Instantaneous)"/1 -> Bus Creator/3  "P"
  PS-Simulink Converter1/1 -> Bus Creator/2, "Power (3ph, Instantaneous)"/2  "i"
  PS-Simulink Converter/1 -> Bus Creator/1, "Power (3ph, Instantaneous)"/1  "v_PhN"
  connections:
  Current Sensor/LConn1 -- In/RConn1
  Out/RConn1 -- Current Sensor/RConn2 -- Phase Voltage Sensor/LConn1
  Grounded Neutral/LConn1 -- Phase Voltage Sensor/RConn2
  PS-Simulink Converter1/LConn1 -- Current Sensor/RConn1
  PS-Simulink Converter/LConn1 -- Phase Voltage Sensor/RConn1

== system A3VSM390/VIPQ Meas0 ==
  note: 2
  Bus Creator : BusCreator  Inputs=4
  Current Sensor : ee_lib/Sensors & Transducers/Current Sensor (Three-Phase)
  Grounded Neutral : ee_lib/Connectors & References/Grounded Neutral (Three-Phase)
  PS-Simulink Converter : nesl_utility/PS-Simulink Converter  PhysicalDomain=network_engine_domain  SubClassName=ps_output  LeftPortType=input  RightPortType=output  PseudoPeriodic=off  Frequencies=[]  VectorFormat=1-D array  Unit=1  AffineConversion=off
  PS-Simulink Converter1 : nesl_utility/PS-Simulink Converter  PhysicalDomain=network_engine_domain  SubClassName=ps_output  LeftPortType=input  RightPortType=output  PseudoPeriodic=off  Frequencies=[]  VectorFormat=1-D array  Unit=1  AffineConversion=off
  Phase Voltage Sensor : ee_lib/Sensors & Transducers/Phase Voltage Sensor (Three-Phase)
  "Power (3ph, Instantaneous)" : spsPower3phInstantaneousLib/Power (3ph, Instantaneous)
  In : PMIOPort  Side=Left
  Out : PMIOPort  Port=2  Side=Right
  meas : Outport  VectorParamsAs1DForOutWhenUnconnected=off
  wires:
  Bus Creator/1 -> meas/1
  "Power (3ph, Instantaneous)"/2 -> Bus Creator/4  "Q"
  "Power (3ph, Instantaneous)"/1 -> Bus Creator/3  "P"
  PS-Simulink Converter1/1 -> Bus Creator/2, "Power (3ph, Instantaneous)"/2  "i"
  PS-Simulink Converter/1 -> Bus Creator/1, "Power (3ph, Instantaneous)"/1  "v_PhN"
  connections:
  Current Sensor/LConn1 -- In/RConn1
  Out/RConn1 -- Current Sensor/RConn2 -- Phase Voltage Sensor/LConn1
  Grounded Neutral/LConn1 -- Phase Voltage Sensor/RConn2
  PS-Simulink Converter1/LConn1 -- Current Sensor/RConn1
  PS-Simulink Converter/LConn1 -- Phase Voltage Sensor/RConn1

== system A3VSM390/VIPQ Meas1 ==
  note: 2
  Bus Creator : BusCreator  Inputs=4
  Current Sensor : ee_lib/Sensors & Transducers/Current Sensor (Three-Phase)
  Grounded Neutral : ee_lib/Connectors & References/Grounded Neutral (Three-Phase)
  PS-Simulink Converter : nesl_utility/PS-Simulink Converter  PhysicalDomain=network_engine_domain  SubClassName=ps_output  LeftPortType=input  RightPortType=output  PseudoPeriodic=off  Frequencies=[]  VectorFormat=1-D array  Unit=1  AffineConversion=off
  PS-Simulink Converter1 : nesl_utility/PS-Simulink Converter  PhysicalDomain=network_engine_domain  SubClassName=ps_output  LeftPortType=input  RightPortType=output  PseudoPeriodic=off  Frequencies=[]  VectorFormat=1-D array  Unit=1  AffineConversion=off
  Phase Voltage Sensor : ee_lib/Sensors & Transducers/Phase Voltage Sensor (Three-Phase)
  "Power (3ph, Instantaneous)" : spsPower3phInstantaneousLib/Power (3ph, Instantaneous)
  In : PMIOPort  Side=Left
  Out : PMIOPort  Port=2  Side=Right
  meas : Outport  VectorParamsAs1DForOutWhenUnconnected=off
  wires:
  PS-Simulink Converter/1 -> "Power (3ph, Instantaneous)"/1, Bus Creator/1  "v_PhN"
  PS-Simulink Converter1/1 -> "Power (3ph, Instantaneous)"/2, Bus Creator/2  "i"
  "Power (3ph, Instantaneous)"/1 -> Bus Creator/3  "P"
  "Power (3ph, Instantaneous)"/2 -> Bus Creator/4  "Q"
  Bus Creator/1 -> meas/1
  connections:
  PS-Simulink Converter/LConn1 -- Phase Voltage Sensor/RConn1
  PS-Simulink Converter1/LConn1 -- Current Sensor/RConn1
  Grounded Neutral/LConn1 -- Phase Voltage Sensor/RConn2
  Phase Voltage Sensor/LConn1 -- Current Sensor/RConn2 -- Out/RConn1
  Current Sensor/LConn1 -- In/RConn1

== system A3VSM390/VIPQ Meas2 ==
  note: 2
  Bus Creator : BusCreator  Inputs=4
  Current Sensor : ee_lib/Sensors & Transducers/Current Sensor (Three-Phase)
  Grounded Neutral : ee_lib/Connectors & References/Grounded Neutral (Three-Phase)
  PS-Simulink Converter : nesl_utility/PS-Simulink Converter  PhysicalDomain=network_engine_domain  SubClassName=ps_output  LeftPortType=input  RightPortType=output  PseudoPeriodic=off  Frequencies=[]  VectorFormat=1-D array  Unit=1  AffineConversion=off
  PS-Simulink Converter1 : nesl_utility/PS-Simulink Converter  PhysicalDomain=network_engine_domain  SubClassName=ps_output  LeftPortType=input  RightPortType=output  PseudoPeriodic=off  Frequencies=[]  VectorFormat=1-D array  Unit=1  AffineConversion=off
  Phase Voltage Sensor : ee_lib/Sensors & Transducers/Phase Voltage Sensor (Three-Phase)
  "Power (3ph, Instantaneous)" : spsPower3phInstantaneousLib/Power (3ph, Instantaneous)
  In : PMIOPort  Side=Left
  Out : PMIOPort  Port=2  Side=Right
  meas : Outport  VectorParamsAs1DForOutWhenUnconnected=off
  wires:
  Bus Creator/1 -> meas/1
  "Power (3ph, Instantaneous)"/2 -> Bus Creator/4  "Q"
  "Power (3ph, Instantaneous)"/1 -> Bus Creator/3  "P"
  PS-Simulink Converter1/1 -> Bus Creator/2, "Power (3ph, Instantaneous)"/2  "i"
  PS-Simulink Converter/1 -> Bus Creator/1, "Power (3ph, Instantaneous)"/1  "v_PhN"
  connections:
  Current Sensor/LConn1 -- In/RConn1
  Out/RConn1 -- Current Sensor/RConn2 -- Phase Voltage Sensor/LConn1
  Grounded Neutral/LConn1 -- Phase Voltage Sensor/RConn2
  PS-Simulink Converter1/LConn1 -- Current Sensor/RConn1
  PS-Simulink Converter/LConn1 -- Phase Voltage Sensor/RConn1

== system A3VSM390/VIPQ Meas5 ==
  note: 2
  Bus Creator : BusCreator  Inputs=4
  Current Sensor : ee_lib/Sensors & Transducers/Current Sensor (Three-Phase)
  Grounded Neutral : ee_lib/Connectors & References/Grounded Neutral (Three-Phase)
  PS-Simulink Converter : nesl_utility/PS-Simulink Converter  PhysicalDomain=network_engine_domain  SubClassName=ps_output  LeftPortType=input  RightPortType=output  PseudoPeriodic=off  Frequencies=[]  VectorFormat=1-D array  Unit=1  AffineConversion=off
  PS-Simulink Converter1 : nesl_utility/PS-Simulink Converter  PhysicalDomain=network_engine_domain  SubClassName=ps_output  LeftPortType=input  RightPortType=output  PseudoPeriodic=off  Frequencies=[]  VectorFormat=1-D array  Unit=1  AffineConversion=off
  Phase Voltage Sensor : ee_lib/Sensors & Transducers/Phase Voltage Sensor (Three-Phase)
  "Power (3ph, Instantaneous)" : spsPower3phInstantaneousLib/Power (3ph, Instantaneous)
  In : PMIOPort  Side=Left
  Out : PMIOPort  Port=2  Side=Right
  meas : Outport  VectorParamsAs1DForOutWhenUnconnected=off
  wires:
  Bus Creator/1 -> meas/1
  "Power (3ph, Instantaneous)"/2 -> Bus Creator/4  "Q"
  "Power (3ph, Instantaneous)"/1 -> Bus Creator/3  "P"
  PS-Simulink Converter1/1 -> Bus Creator/2, "Power (3ph, Instantaneous)"/2  "i"
  PS-Simulink Converter/1 -> Bus Creator/1, "Power (3ph, Instantaneous)"/1  "v_PhN"
  connections:
  Current Sensor/LConn1 -- In/RConn1
  Out/RConn1 -- Current Sensor/RConn2 -- Phase Voltage Sensor/LConn1
  Grounded Neutral/LConn1 -- Phase Voltage Sensor/RConn2
  PS-Simulink Converter1/LConn1 -- Current Sensor/RConn1
  PS-Simulink Converter/LConn1 -- Phase Voltage Sensor/RConn1
